simulink model "Test_Byte_Multiplexer_2_to_1"  (R2023a)
settings: Solver=ode45  StartTime=0.0  StopTime=len  RelTol=1e-3  EnableMultiTasking=on
libraries: Miscellaneous x3, Byte_Multiplexers_Lib x1, simulink x1
settings Model: Creator=N  LastModifiedBy=Jozko Mrkvicka
settings SolverCC: AlgebraicLoopSolver=TrustRegion
settings DataIOCC: SaveFormat=Array  ReturnWorkspaceOutputs=off
settings OptimizationCC: LifeSpan=inf
settings DebuggingCC: UnconnectedInputMsg=warning  UnconnectedOutputMsg=warning  UnconnectedLineMsg=warning  SFUnexpectedBacktrackingDiag=warning  SFNoUnconditionalDefaultTransitionDiag=warning  SFExecutionAtInitializationDiag=none  ArithmeticOperatorsInVariantConditions=warning
settings HardwareCC: ProdWordSize=32
settings SFSimCC: SimUseLocalCustomCode=off  CustomCodeUndefinedFunction=UseInterfaceOnly
settings RTWCC: RTWUseLocalCustomCode=off
settings CodeAppCC: StateflowObjectComments=on
settings GRTTargetCC: TargetLangStandard=C89/C90 (ANSI)
settings ConfigComp: CovMetricSettings=dw  CovSaveCumulativeToWorkspaceVar=on  CovSaveSingleToWorkspaceVar=on  CovExternalEMLEnable=off

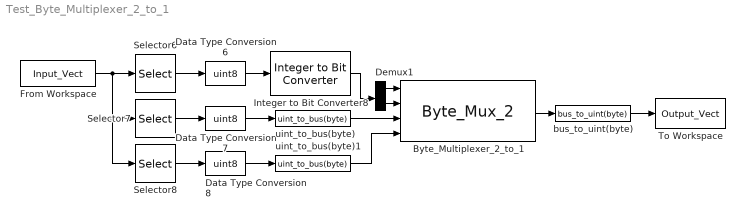
== system Test_Byte_Multiplexer_2_to_1 ==
  Byte_Multiplexer_2_to_1 : Byte_Multiplexers_Lib/Byte_Mux_2  SystemSampleTime=-1  VariantActivationTime=update diagram  Latency=0  AutoFrameSizeCalculation=off
  Data Type Conversion6 : DataTypeConversion  OutDataTypeStr=uint8  SaturateOnIntegerOverflow=off  RndMeth=Floor
  Data Type Conversion7 : DataTypeConversion  OutDataTypeStr=uint8  SaturateOnIntegerOverflow=off  RndMeth=Floor
  Data Type Conversion8 : DataTypeConversion  OutDataTypeStr=uint8  SaturateOnIntegerOverflow=off  RndMeth=Floor
  Demux1 : Demux  Outputs=2
  From Workspace : FromWorkspace  VariableName=Input_Vect  SampleTime=1  Interpolate=off  ZeroCross=off  OutputAfterFinalValue=Holding final value
  Integer to Bit Converter8 : simulink/Logic and Bit Operations/Integer to Bit Converter  nbits=2  signedInputValues=Unsigned  bitOrder=MSB first  outDtype=boolean
      settings: LibrarySourceBlock=|
      | commutil2/Integer to Bit
      | Converter
  Selector6 : Selector  IndexMode=Zero-based  InputPortWidth=3  SampleTime=1  IndexOptions=Index vector (dialog)  Indices=0  OutputSizes=1
  Selector7 : Selector  IndexMode=Zero-based  InputPortWidth=3  IndexOptions=Index vector (dialog)  Indices=1  OutputSizes=1
  Selector8 : Selector  IndexMode=Zero-based  InputPortWidth=3  IndexOptions=Index vector (dialog)  Indices=2  OutputSizes=1
  To Workspace : ToWorkspace  VariableName=Output_Vect  SampleTime=1
  bus_to_uint(byte) : Miscellaneous/bus_to_uint(byte)  SystemSampleTime=-1  VariantActivationTime=update diagram  Latency=0  AutoFrameSizeCalculation=off
  uint_to_bus(byte) : Miscellaneous/uint_to_bus(byte)  SystemSampleTime=-1  VariantActivationTime=update diagram  Latency=0  AutoFrameSizeCalculation=off
  uint_to_bus(byte)1 : Miscellaneous/uint_to_bus(byte)  SystemSampleTime=-1  VariantActivationTime=update diagram  Latency=0  AutoFrameSizeCalculation=off
  wires:
  Data Type Conversion7/1 -> uint_to_bus(byte)/1
  uint_to_bus(byte)1/1 -> Byte_Multiplexer_2_to_1/4
  Byte_Multiplexer_2_to_1/1 -> bus_to_uint(byte)/1
  Integer to Bit Converter8/1 -> Demux1/1
  Selector6/1 -> Data Type Conversion6/1
  Selector7/1 -> Data Type Conversion7/1
  Data Type Conversion6/1 -> Integer to Bit Converter8/1
  From Workspace/1 -> Selector8/1, Selector7/1, Selector6/1
  Selector8/1 -> Data Type Conversion8/1
  Demux1/1 -> Byte_Multiplexer_2_to_1/1
  Demux1/2 -> Byte_Multiplexer_2_to_1/2
  uint_to_bus(byte)/1 -> Byte_Multiplexer_2_to_1/3
  Data Type Conversion8/1 -> uint_to_bus(byte)1/1
  bus_to_uint(byte)/1 -> To Workspace/1
